simulink model "udpcommsdemo"  (R2016a)
settings: Solver=VariableStepAuto  StartTime=0.0  StopTime=10.0  RelTol=1e-3
undefined symbols (not defined in the file): sldrtexcb_modeswitch, Standard_Devices, UDP_Protocol
libraries: sldrtlib x4, simulink x1
settings Model: Creator=julianleland  LastModifiedBy=julianleland

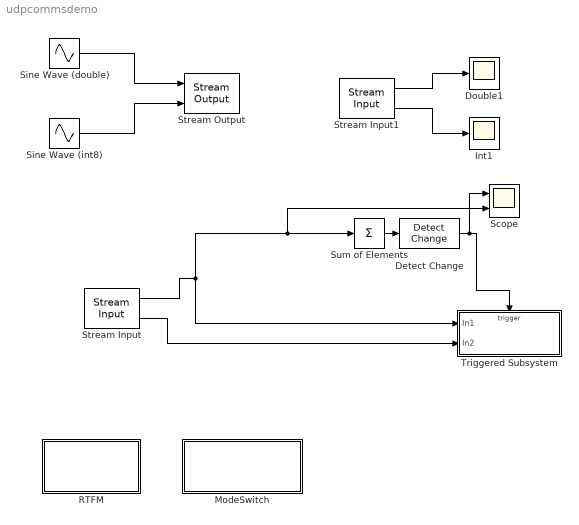
== system udpcommsdemo ==
  Detect Change : simulink/Logic and Bit Operations/Detect Change  vinit=0  OutDataTypeStr=boolean
  Double1 : Scope
  Int1 : Scope
  ModeSwitch : Subsystem  InitFcn=sldrtexcb_modeswitch('CheckKernel');  mask(Simulink Desktop Real-Time Example Mode Switch){}
      settings: OpenFcn=sldrtexcb_modeswitch(gcbh);
      mask Display: disp('Switch To\nExternal Mode');
  "RTFM " : Subsystem  mask(Simulink Desktop Real-Time Example Info){}
      settings: OpenFcn=web([docroot '/rtwin/examples/stream-input-output.html']);
      mask Display: disp('Info')
  Scope : Scope  NumInputPorts=2
  Sine Wave (double) : Sin  Amplitude=1:4  Frequency=2  SampleTime=0
  Sine Wave (int8) : Sin  Amplitude=1:8  Frequency=2  SampleTime=0
  Stream Input : sldrtlib/Stream Input  SampleTime=0.025  MaxMissedTicks=50  ShowMissedTicks=off  YieldWhenWaiting=off  DrvName=Standard_Devices/UDP_Protocol  DrvAddress=36880  DrvOptions=[2130706433 36864]  DataTypes={'4*double', '8*int8'}  FormatString='%f %f %f %f %d %d %d %d %d %d %d %d'  Terminator={ '\r', '\n' }  ShowReady=off  ShowError=off
      settings: AttributesFormatString=Standard Devices\nUDP Protocol [9010h]
  Stream Input1 : sldrtlib/Stream Input  SampleTime=0.01  MaxMissedTicks=50  ShowMissedTicks=off  YieldWhenWaiting=off  DrvName=Standard_Devices/UDP_Protocol  DrvAddress=12000  DrvOptions=[2130706433 12001]  DataTypes={'4*double', '8*int8'}  FormatString='%f %f %f %f %d %d %d %d %d %d %d %d'  Terminator={ '\r', '\n' }  ShowReady=off  ShowError=off
      settings: AttributesFormatString=Standard Devices\nUDP Protocol [2EE0h]
  Stream Output : sldrtlib/Stream Output  SampleTime=0.5  MaxMissedTicks=50  ShowMissedTicks=off  YieldWhenWaiting=off  DrvName=Standard_Devices/UDP_Protocol  DrvAddress=36864  DrvOptions=[2130706433 36880]  PortSizes=[4 8]  FormatString='%g %g %g %g %d %d %d %d %d %d %d %d\n'  ShowReady=off  ShowError=off  InitialValue=[]  FinalValue=[]
      settings: AttributesFormatString=Standard Devices\nUDP Protocol [9000h]
  Sum of Elements : Sum  Inputs=+
  Triggered Subsystem : Subsystem  TreatAsAtomicUnit=on
  wires:
  Sine Wave (int8)/1 -> Stream Output/2
  Sine Wave (double)/1 -> Stream Output/1
  Stream Input1/1 -> Double1/1
  Stream Input1/2 -> Int1/1
  Stream Input/1 -> Triggered Subsystem/1(In1), Sum of Elements/1, Scope/2
  Sum of Elements/1 -> Detect Change/1
  Stream Input/2 -> Triggered Subsystem/2(In2)
  Detect Change/1 -> Scope/1, Triggered Subsystem/Trigger

== system udpcommsdemo/ModeSwitch ==

== system udpcommsdemo/RTFM  ==

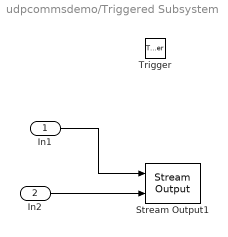
== system udpcommsdemo/Triggered Subsystem ==
  In1 : Inport
  In2 : Inport  Port=2
  Trigger : TriggerPort  VariantControl=Variant  StatesWhenEnabling=reset
  Stream Output1 : sldrtlib/Stream Output  SampleTime=inf  MaxMissedTicks=50  ShowMissedTicks=off  YieldWhenWaiting=off  DrvName=Standard_Devices/UDP_Protocol  DrvAddress=12001  DrvOptions=[2130706433 12000]  PortSizes=[4 8]  FormatString='%g %g %g %g %d %d %d %d %d %d %d %d\n'  ShowReady=off  ShowError=off  InitialValue=[]  FinalValue=[]
      settings: AttributesFormatString=Standard Devices\nUDP Protocol [2EE1h]
  wires:
  In1/1 -> Stream Output1/1
  In2/1 -> Stream Output1/2
